simulink model "topic1"  (R2019b)
settings: Solver=VariableStepAuto  StartTime=0.0  StopTime=0.06  RelTol=1e-3
libraries: powerlib x22, powerlib_meascontrol x7
settings Model: Creator=96547  LastModifiedBy=96547

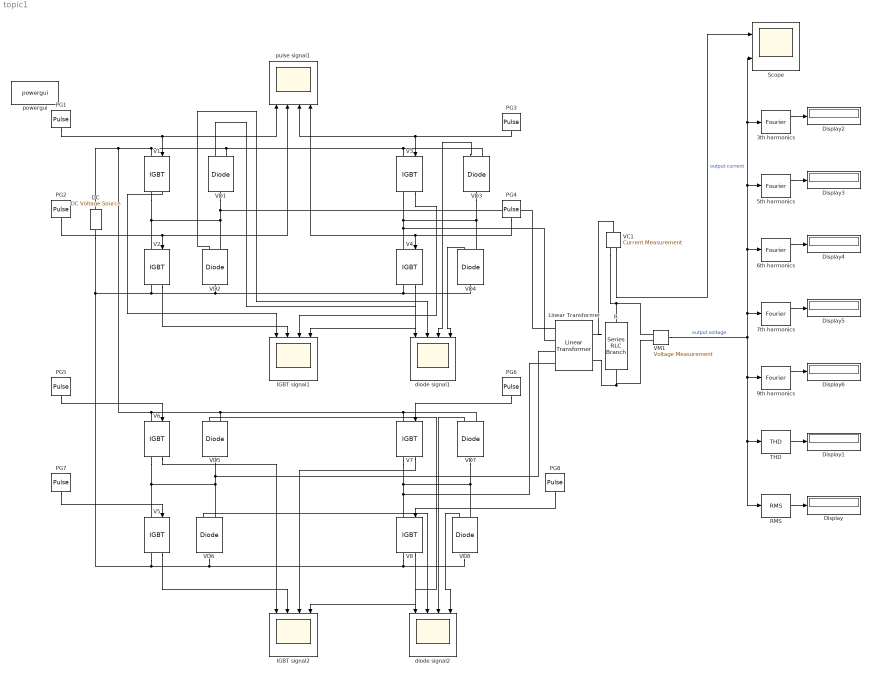
== system topic1 ==
  3th harmonics : powerlib_meascontrol/Measurements/Fourier  Freq=50  n=3  InInit=[0, 0]  Ts=0
      settings: SourceProductName=Simscape Electrical
  5th harmonics : powerlib_meascontrol/Measurements/Fourier  Freq=50  n=5  InInit=[0, 0]  Ts=0
      settings: SourceProductName=Simscape Electrical
  6th harmonics : powerlib_meascontrol/Measurements/Fourier  Freq=50  n=6  InInit=[0, 0]  Ts=0
      settings: SourceProductName=Simscape Electrical
  7th harmonics : powerlib_meascontrol/Measurements/Fourier  Freq=50  n=7  InInit=[0, 0]  Ts=0
      settings: SourceProductName=Simscape Electrical
  9th harmonics : powerlib_meascontrol/Measurements/Fourier  Freq=50  n=9  InInit=[0, 0]  Ts=0
      settings: SourceProductName=Simscape Electrical
  DC : powerlib/Electrical Sources/DC Voltage Source  Amplitude=400  Measurements=None
      settings: SourceProductName=Simscape Electrical
  Display{,1..6} (7 alike) : Display
  IGBT signal1 : Scope  NumInputPorts=4
  IGBT signal2 : Scope  NumInputPorts=4
  Linear Transformer : powerlib/Elements/Linear Transformer  UNITS=pu  NominalPower=[ 250e6 50 ]  winding1="[ 735e3  0  0 ]"  winding2="[ 315e3  0  0 ]"  ThreeWindings=on  winding3="[ 315e3  0  0 ]"  RmLm=[ 500 500 ]  Measurements=None  DataType=off
      settings: SourceProductName=Simscape Electrical
  PG1 : DiscretePulseGenerator  PulseType=Time based  Period=0.02  PulseWidth=50
  PG2 : DiscretePulseGenerator  PulseType=Time based  Period=0.02  PulseWidth=50  PhaseDelay=0.01
  PG3 : DiscretePulseGenerator  PulseType=Time based  Period=0.02  PulseWidth=50  PhaseDelay=0.02*(1/6)
  PG4 : DiscretePulseGenerator  PulseType=Time based  Period=0.02  PulseWidth=50  PhaseDelay=0.01+0.02*(1/6)
  PG5 : DiscretePulseGenerator  PulseType=Time based  Period=0.02  PulseWidth=50
  PG6 : DiscretePulseGenerator  PulseType=Time based  Period=0.02  PulseWidth=50  PhaseDelay=0.02*(1/6)
  PG7 : DiscretePulseGenerator  PulseType=Time based  Period=0.02  PulseWidth=50  PhaseDelay=0.01
  PG8 : DiscretePulseGenerator  PulseType=Time based  Period=0.02  PulseWidth=20  PhaseDelay=0.02*(1/6)+1
  R : powerlib/Elements/Series RLC Branch  LConnTagsString=__new0  RConnTagsString=__new0  BranchType=R  Resistance=8  Inductance=1e-3  SetiL0=off  InitialCurrent=0  Capacitance=1e-6  Setx0=off  InitialVoltage=0  Measurements=None
      settings: SourceProductName=Simscape Electrical
  RMS : powerlib_meascontrol/Measurements/RMS  TrueRMS=on  Freq=60  RMSInit=120  Ts=0
      settings: SourceProductName=Simscape Electrical
  Scope : Scope  NumInputPorts=2
  THD : powerlib_meascontrol/Measurements/THD  Freq=60  Ts=0
      settings: SourceProductName=Simscape Electrical
  V{1..8} (8 alike) : powerlib/Power Electronics/IGBT  Ron=0.001  Lon=0  Vf=1  Tf=1e-6  Tt=2e-6  IC=0  Rs=1e5  Cs=inf  Measurements=on
      settings: SourceProductName=Simscape Electrical
  VC1 : powerlib/Measurements/Current Measurement  PhasorSimulation=off  OutputType=Complex  PSBequivalent=0
      settings: SourceProductName=Simscape Electrical
  VD{1..8} (8 alike) : powerlib/Power Electronics/Diode  Ron=0.001  Lon=0  Vf=0.8  IC=0  UseSnubber=0  Rs=500  Cs=250e-9  Measurements=on
      settings: SourceProductName=Simscape Electrical
  VM1 : powerlib/Measurements/Voltage Measurement  PhasorSimulation=off  OutputType=Complex  PSBequivalent=0
      settings: SourceProductName=Simscape Electrical
  diode signal1 : Scope  NumInputPorts=4
  diode signal2 : Scope  NumInputPorts=4
  powergui : powerlib/powergui  Priority=1  SimulationMode=Continuous  SampleTime=50e-6  frequency=60  Iterations=50  frequencyindice=0  Pbase=100e6  ErrMax=1e-4  UnitsV=kV  UnitsW=MW  buscounter=0  FunctionMessages=off  echomessages=off  EnableUseOfTLC=off  CurrentSourceSwitches=off  DisableSnubberDevices=off  DisableRonSwitches=off  DisableVfSwitches=off  DisplayEquations=off  AutomaticDiscreteSolvers=off  SolverType=Tustin/Backward Euler (TBE)  Interpol=off  ExternalGateDelay=off  methode=off  Ts=100  x0status=blocks  SPID=on  SwTol=0  HookPort=off  NonlinearTolerance=1e-4  nMaxIteration=100  ContinueOnMaxIteration=off  RestoreLinks=warning  ResistiveCurrentMeasurement=off  Frange=[0:2:500]  Ylog=off  Xlog=on  ShowGrid=off  save=off  variable=ZData  structure=0  ZoomFFT=off  StartTime=0.0  cycles=1  DisplayStyle=1  fundamental=60  FreqAxis=off  MaxFrequency=1000  frequencyindicesteady=1  RmsSteady=1  display=off
      settings: SourceProductName=Simscape Electrical
  pulse signal1 : Scope  NumInputPorts=4
  wires:
  PG3/1 -> V3/1, pulse signal1/3
  PG1/1 -> V1/1, pulse signal1/1
  VM1/1 -> RMS/1, THD/1, 9th harmonics/1, Scope/2, 3th harmonics/1, 5th harmonics/1, 6th harmonics/1, 7th harmonics/1  "output voltage"
  RMS/1 -> Display/1
  THD/1 -> Display1/1
  3th harmonics/1 -> Display2/1
  5th harmonics/1 -> Display3/1
  6th harmonics/1 -> Display4/1
  7th harmonics/1 -> Display5/1
  9th harmonics/1 -> Display6/1
  PG2/1 -> V2/1, pulse signal1/2
  PG4/1 -> V4/1, pulse signal1/4
  PG7/1 -> V5/1
  PG8/1 -> V8/1
  PG5/1 -> V6/1
  PG6/1 -> V7/1
  V1/1 -> IGBT signal1/1
  V2/1 -> IGBT signal1/2
  V3/1 -> IGBT signal1/3
  V4/1 -> IGBT signal1/4
  V6/1 -> IGBT signal2/1
  V5/1 -> IGBT signal2/2
  V7/1 -> IGBT signal2/3
  V8/1 -> IGBT signal2/4
  VD1/1 -> diode signal1/1
  VD2/1 -> diode signal1/2
  VD3/1 -> diode signal1/3
  VD4/1 -> diode signal1/4
  VD5/1 -> diode signal2/1
  VD6/1 -> diode signal2/2
  VD7/1 -> diode signal2/3
  VD8/1 -> diode signal2/4
  VC1/1 -> Scope/1  "output current"
  connections:
  V1/LConn1 -- DC/RConn1 -- VD7/RConn1 -- V7/LConn1 -- VD5/RConn1 -- V6/LConn1 -- VD3/RConn1 -- V3/LConn1 -- VD1/RConn1
  DC/LConn1 -- V5/RConn1 -- VD6/LConn1 -- V8/RConn1 -- VD8/LConn1 -- V2/RConn1 -- VD4/LConn1 -- V4/RConn1 -- VD2/LConn1
  VD1/LConn1 -- VD2/RConn1 -- V1/RConn1 -- V2/LConn1 -- Linear Transformer/RConn4
  V7/RConn1 -- V8/LConn1 -- Linear Transformer/RConn1 -- VD8/RConn1 -- VD7/LConn1
  VM1/LConn1 -- VC1/RConn1 -- R/LConn1
  Linear Transformer/LConn1 -- VM1/LConn2 -- R/RConn1
  VD3/LConn1 -- VD4/RConn1 -- Linear Transformer/RConn3 -- V4/LConn1 -- V3/RConn1
  V6/RConn1 -- V5/LConn1 -- VD6/RConn1 -- VD5/LConn1 -- Linear Transformer/RConn2
  Linear Transformer/LConn2 -- VC1/LConn1
